simulink model "Condensor"  (R2020a)
settings: Solver=VariableStepAuto  StartTime=0.0  StopTime=10.0  RelTol=1e-3
settings Model: Creator=YJT  LastModifiedBy=YJT

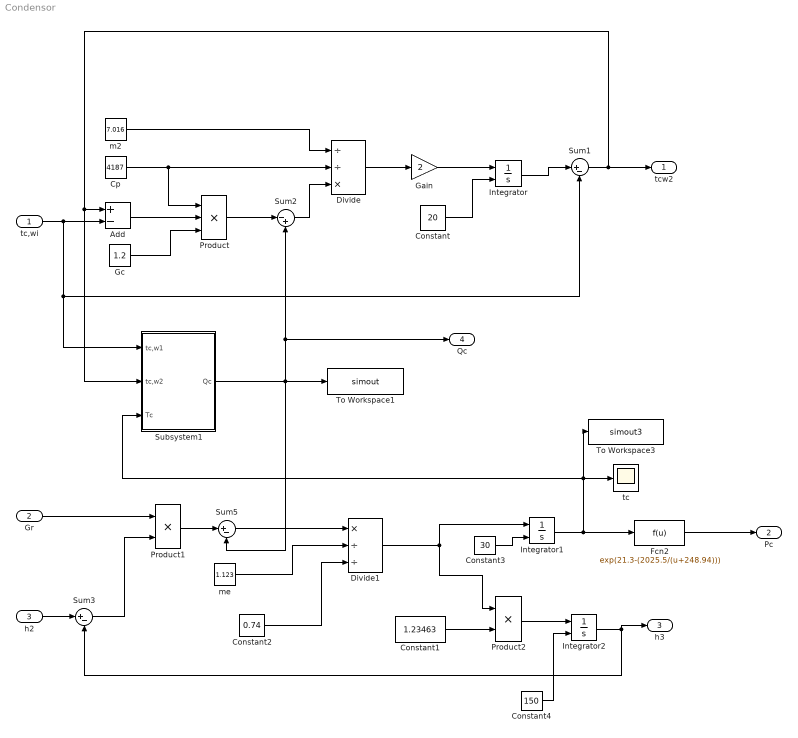
== system Condensor ==
  tc,wi : Inport
  Gr : Inport  Port=2
  h2 : Inport  Port=3
  Add : Sum  Inputs=+-
  Constant : Constant  Value=20
  Constant1 : Constant  Value=1.23463
  Constant2 : Constant  Value=0.74
  Constant3 : Constant  Value=30
  Constant4 : Constant  Value=150
  Cp : Constant  Value=4187
  Divide : Product  Inputs=//*
  Divide1 : Product  Inputs=*//
  Fcn2 : Fcn  Expr=exp(21.3-(2025.5/(u+248.94)))
  Gain : Gain  Gain=2
  Gc : Constant  Value=1.2
  Integrator : Integrator  InitialConditionSource=external
  Integrator1 : Integrator  InitialConditionSource=external
  Integrator2 : Integrator  InitialConditionSource=external
  Product : Product  Inputs=3
  Product1 : Product
  Product2 : Product
  Subsystem1 : Subsystem
  Sum1 : Sum  Inputs=|+-
  Sum2 : Sum  Inputs=|-+
  Sum3 : Sum  Inputs=|+-
  Sum5 : Sum  Inputs=|+-
  To Workspace1 : ToWorkspace  VariableName=simout  SaveFormat=Timeseries  SampleTime=-1
  To Workspace3 : ToWorkspace  VariableName=simout3  SaveFormat=Timeseries  SampleTime=-1
  m2 : Constant  Value=7.016
  me : Constant  Value=1.123
  tc : Scope
  tcw2 : Outport
  Pc : Outport  Port=2
  h3 : Outport  Port=3
  Qc : Outport  Port=4
  wires:
  Integrator1/1 -> Subsystem1/3(Tc), tc/1, To Workspace3/1, Fcn2/1
  Sum2/1 -> Divide/3
  Cp/1 -> Product/1, Divide/2
  Divide/1 -> Gain/1
  Constant2/1 -> Divide1/3
  Divide1/1 -> Integrator1/1, Product2/1
  Add/1 -> Product/2
  me/1 -> Divide1/2
  Subsystem1/1(Qc) -> Sum5/2, Sum2/2, Qc/1, To Workspace1/1
  Product/1 -> Sum2/1
  Gc/1 -> Product/3
  Sum5/1 -> Divide1/1
  Gain/1 -> Integrator/1
  Fcn2/1 -> Pc/1
  Integrator/1 -> Sum1/1
  Constant4/1 -> Integrator2/2
  Sum1/1 -> Subsystem1/2(tc,w2), Add/1, tcw2/1
  Product2/1 -> Integrator2/1
  Constant3/1 -> Integrator1/2
  Sum3/1 -> Product1/2
  m2/1 -> Divide/1
  Constant1/1 -> Product2/2
  h2/1 -> Sum3/1
  tc,wi/1 -> Add/2, Subsystem1/1(tc,w1), Sum1/2
  Gr/1 -> Product1/1
  Constant/1 -> Integrator/2
  Integrator2/1 -> h3/1, Sum3/2
  Product1/1 -> Sum5/1

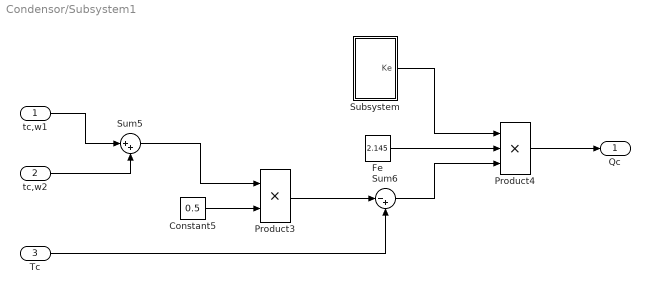
== system Condensor/Subsystem1 ==
  tc,w1 : Inport
  tc,w2 : Inport  Port=2
  Tc : Inport  Port=3
  Constant5 : Constant  Value=0.5
  Fe : Constant  Value=2.145
  Product3 : Product
  Product4 : Product  Inputs=3
  Subsystem : Subsystem
  Sum5 : Sum  Inputs=|++
  Sum6 : Sum  Inputs=|-+
  Qc : Outport
  wires:
  Product4/1 -> Qc/1
  Subsystem/1(Ke) -> Product4/1
  tc,w2/1 -> Sum5/2
  Product3/1 -> Sum6/1
  Fe/1 -> Product4/2
  Sum6/1 -> Product4/3
  Tc/1 -> Sum6/2
  Constant5/1 -> Product3/2
  Sum5/1 -> Product3/1
  tc,w1/1 -> Sum5/1

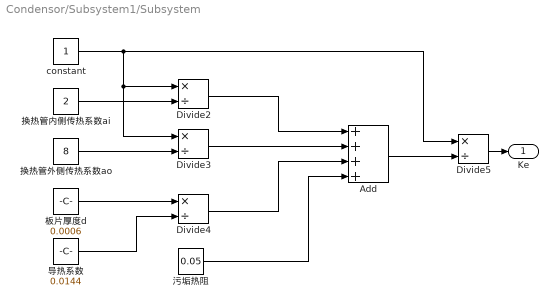
== system Condensor/Subsystem1/Subsystem ==
  Add : Sum  Inputs=++++
  Divide{2..5} (4 alike) : Product  Inputs=*/
  constant : Constant
  导热系数 : Constant  Value=0.0144
  换热管内侧传热系数ai : Constant  Value=2
  换热管外侧传热系数ao : Constant  Value=8
  板片厚度d : Constant  Value=0.0006
  污垢热阻 : Constant  Value=0.05
  Ke : Outport
  wires:
  constant/1 -> Divide5/1, Divide2/1, Divide3/1
  导热系数/1 -> Divide4/2
  Divide3/1 -> Add/2
  污垢热阻/1 -> Add/4
  换热管内侧传热系数ai/1 -> Divide2/2
  板片厚度d/1 -> Divide4/1
  Divide2/1 -> Add/1
  换热管外侧传热系数ao/1 -> Divide3/2
  Add/1 -> Divide5/2
  Divide4/1 -> Add/3
  Divide5/1 -> Ke/1
